simulink model "P8_Signal_Conditioning_Circuit"  (R2023b)
settings: Solver=FixedStepAuto  StartTime=0.0  StopTime=1  FixedStep=1e-6  RelTol=1e-9
libraries: spsSeriesRLCBranchLib x23, spsVoltageMeasurementLib x15, spsGroundLib x14, spsDiodeLib x9, spsControlledVoltageSourceLib x5, simulink x4, spsACVoltageSourceLib x2, spsIdealSwitchLib x1, eePwmGenerator x1, spsDCVoltageSourceLib x1, sps_lib x1
settings Model: Creator=Lucas  LastModifiedBy=Lucas

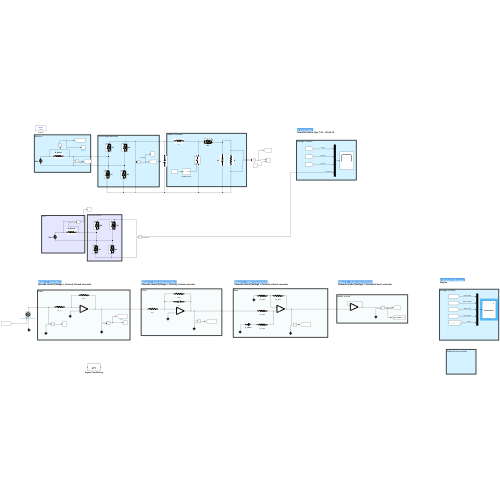
[thumbnail: Simulink's stored preview of the top-level diagram]
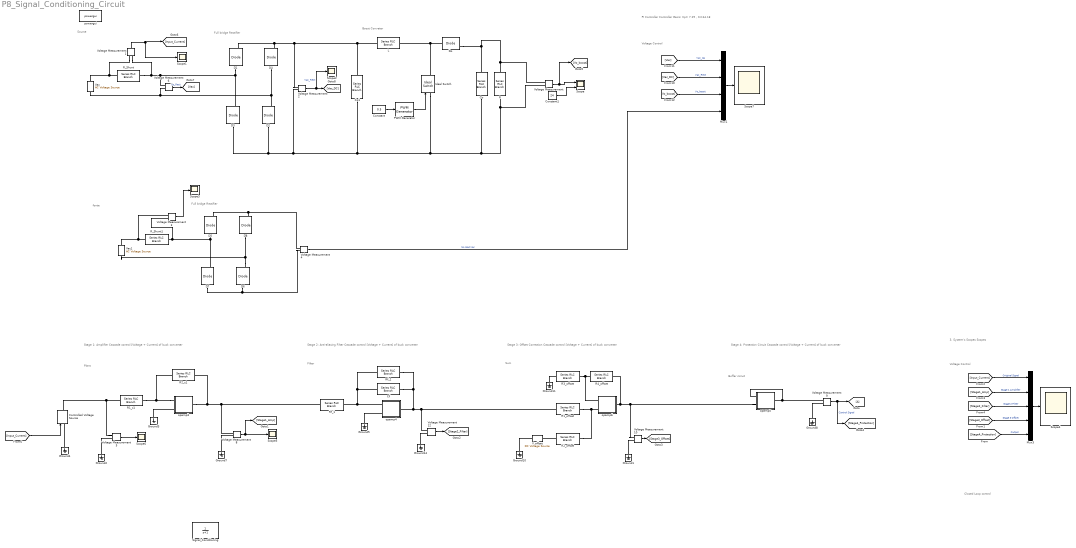
== system P8_Signal_Conditioning_Circuit ==
  note: Boost Conveter
  note: Full bridge Rectifier
  note: Source
  note: Full bridge Rectifier
  note: fonte
  note: PI Controller
      | Controller Gains: Kp= 7.29 , Ki=44.18
  note: Stage 1: Amplifier
      | Cascade control [Voltage + Current] of buck converter
  note: Stage 2: Anti-aliasing Filter
      | Cascade control [Voltage + Current] of buck converter
  note: Stage 3: Offset Correction
      | Cascade control [Voltage + Current] of buck converter
  note: Stage 4: Protection Circuit
      | Cascade control [Voltage + Current] of buck converter
  note: Closed Loop control
  note: Plant
  note: Voltage Control
  note: 3. System's Scopes
      | Scopes
  note: Filter
  note: Sum
  note: Buffer circuit
  note: Voltage Control
  Cf : spsSeriesRLCBranchLib/Series RLC Branch  LConnTagsString=__new0  RConnTagsString=__new0  BranchType=C  Resistance=1e3  Inductance=1e-3  SetiL0=off  InitialCurrent=0  Capacitance=4.9e-9  Setx0=off  InitialVoltage=0  Measurements=None
  Co : spsSeriesRLCBranchLib/Series RLC Branch  LConnTagsString=__new0  RConnTagsString=__new0  BranchType=C  Resistance=1  Inductance=1e-3  SetiL0=off  InitialCurrent=0  Capacitance=510e-6  Setx0=off  InitialVoltage=0  Measurements=None
  Co1 : spsSeriesRLCBranchLib/Series RLC Branch  LConnTagsString=__new0  RConnTagsString=__new0  BranchType=C  Resistance=1  Inductance=1e-3  SetiL0=off  InitialCurrent=0  Capacitance=1  Setx0=off  InitialVoltage=0  Measurements=None
  Constant : Constant  Value=0.5
  Constant1 : Constant  Value=24
  Controlled Voltage Source : spsControlledVoltageSourceLib/Controlled Voltage Source  Initialize=on  Source_Type=AC  Amplitude=0  Phase=0  Frequency=0  Measurements=None
  D{1..8} (8 alike) : spsDiodeLib/Diode  Ron=0.001  Lon=0  Vf=0  IC=0  UseSnubber=0  Rs=500  Cs=250e-9  Measurements=on
  Do : spsDiodeLib/Diode  Ron=0.001  Lon=0  Vf=0  IC=0  UseSnubber=0  Rs=500  Cs=250e-9  Measurements=on
  Goto : Goto
  Ground{1..5,7..8,10..11,14} (10 alike) : spsGroundLib/Ground  LConnTagsString=a
  Ideal Switch : spsIdealSwitchLib/Ideal Switch  Ron=0.001  Lon=0  IC=0  Rs=inf  Cs=inf  Measurements=on
  L : spsSeriesRLCBranchLib/Series RLC Branch  LConnTagsString=__new0  RConnTagsString=__new0  BranchType=L  Resistance=1  Inductance=100e-3  SetiL0=off  InitialCurrent=0  Capacitance=1e-6  Setx0=off  InitialVoltage=0  Measurements=None
  Mux1 : Mux
  Mux3 : Mux  Inputs=5
  PWM Generator : eePwmGenerator/PWM Generator  CarrCount=Up  Tper=1/(80e3)  Tdelay=0  Ts=1e-6
  R : spsSeriesRLCBranchLib/Series RLC Branch  LConnTagsString=__new0  RConnTagsString=__new0  BranchType=R  Resistance=10  Inductance=1e-3  SetiL0=off  InitialCurrent=0  Capacitance=1e-6  Setx0=off  InitialVoltage=0  Measurements=None
  R1_c1 : spsSeriesRLCBranchLib/Series RLC Branch  LConnTagsString=__new0  RConnTagsString=__new0  BranchType=R  Resistance=4e3  Inductance=1e-3  SetiL0=off  InitialCurrent=0  Capacitance=1e-6  Setx0=off  InitialVoltage=0  Measurements=None
  R1_offset : spsSeriesRLCBranchLib/Series RLC Branch  LConnTagsString=__new0  RConnTagsString=__new0  BranchType=R  Resistance=10e3  Inductance=1e-3  SetiL0=off  InitialCurrent=0  Capacitance=1e-6  Setx0=off  InitialVoltage=0  Measurements=None
  R2_c1 : spsSeriesRLCBranchLib/Series RLC Branch  LConnTagsString=__new0  RConnTagsString=__new0  BranchType=R  Resistance=1e3  Inductance=1e-3  SetiL0=off  InitialCurrent=0  Capacitance=1e-6  Setx0=off  InitialVoltage=0  Measurements=None
  R2_offset : spsSeriesRLCBranchLib/Series RLC Branch  LConnTagsString=__new0  RConnTagsString=__new0  BranchType=R  Resistance=10e3  Inductance=1e-3  SetiL0=off  InitialCurrent=0  Capacitance=1e-6  Setx0=off  InitialVoltage=0  Measurements=None
  R3_offset : spsSeriesRLCBranchLib/Series RLC Branch  LConnTagsString=__new0  RConnTagsString=__new0  BranchType=R  Resistance=10e3  Inductance=1e-3  SetiL0=off  InitialCurrent=0  Capacitance=1e-6  Setx0=off  InitialVoltage=0  Measurements=None
  R4_offset : spsSeriesRLCBranchLib/Series RLC Branch  LConnTagsString=__new0  RConnTagsString=__new0  BranchType=R  Resistance=10e3  Inductance=1e-3  SetiL0=off  InitialCurrent=0  Capacitance=1e-6  Setx0=off  InitialVoltage=0  Measurements=None
  R_Shunt : spsSeriesRLCBranchLib/Series RLC Branch  LConnTagsString=__new0  RConnTagsString=__new0  BranchType=R  Resistance=0.1  Inductance=1e-3  SetiL0=off  InitialCurrent=0  Capacitance=1e-6  Setx0=off  InitialVoltage=0  Measurements=None
  R_Shunt1 : spsSeriesRLCBranchLib/Series RLC Branch  LConnTagsString=__new0  RConnTagsString=__new0  BranchType=R  Resistance=0.1  Inductance=1e-3  SetiL0=off  InitialCurrent=0  Capacitance=1e-6  Setx0=off  InitialVoltage=0  Measurements=None
  Rf_1 : spsSeriesRLCBranchLib/Series RLC Branch  LConnTagsString=__new0  RConnTagsString=__new0  BranchType=R  Resistance=1e3  Inductance=1e-3  SetiL0=off  InitialCurrent=0  Capacitance=1e-6  Setx0=off  InitialVoltage=0  Measurements=None
  Rf_2 : spsSeriesRLCBranchLib/Series RLC Branch  LConnTagsString=__new0  RConnTagsString=__new0  BranchType=R  Resistance=1e3  Inductance=1e-3  SetiL0=off  InitialCurrent=0  Capacitance=1e-6  Setx0=off  InitialVoltage=0  Measurements=None
  Scope : Scope  NumInputPorts=2
  Scope{1..7} (7 alike) : Scope
  Signal_Conditioning : TransferFcn  Denominator=[1 1]
  V_offset : spsDCVoltageSourceLib/DC Voltage Source  Amplitude=2.5  Measurements=None
  Vac : spsACVoltageSourceLib/AC Voltage Source  Amplitude=12  Phase=0  Frequency=60  SampleTime=1e-6  Measurements=None  BusType=swing  Pref=10e3  Qref=0  Qmin=-inf  Qmax=+inf
  Vac1 : spsACVoltageSourceLib/AC Voltage Source  Amplitude=12  Phase=0  Frequency=60  SampleTime=0  Measurements=None  BusType=swing  Pref=10e3  Qref=0  Qmin=-inf  Qmax=+inf
  Voltage Measurement{,1..6,8..10,12} (11 alike) : spsVoltageMeasurementLib/Voltage Measurement  PhasorSimulation=off  OutputType=Complex  PSBequivalent=0
  opamp3 : Subsystem  mask(Opamp){Ri=1e7, Ro=100, A=200000, U1=15, U2=-15}
      mask prompts: Ri "Input Resistance"; Ro "Output Resistance"; A "Open loop amplification"; U1 "Upper limit supply voltage"; U2 "Lower limit supply voltage"
      mask Display:
      | plot([10 20 30 40], [10 12 14 16],[10 20 30 40], [22 20 18 16],[10 10],[10 22])
      | text(10,13.4,'+')
      | text(10,21,'_')
  opamp4 : Subsystem  mask(Opamp){Ri=1e7, Ro=100, A=200000, U1=15, U2=-15}
      mask prompts: Ri "Input Resistance"; Ro "Output Resistance"; A "Open loop amplification"; U1 "Upper limit supply voltage"; U2 "Lower limit supply voltage"
      mask Display:
      | plot([10 20 30 40], [10 12 14 16],[10 20 30 40], [22 20 18 16],[10 10],[10 22])
      | text(10,13.4,'+')
      | text(10,21,'_')
  opamp5 : Subsystem  mask(Opamp){Ri=1e7, Ro=100, A=200000, U1=5, U2=0}
      mask prompts: Ri "Input Resistance"; Ro "Output Resistance"; A "Open loop amplification"; U1 "Upper limit supply voltage"; U2 "Lower limit supply voltage"
      mask Display:
      | plot([10 20 30 40], [10 12 14 16],[10 20 30 40], [22 20 18 16],[10 10],[10 22])
      | text(10,13.4,'+')
      | text(10,21,'_')
  opamp6 : Subsystem  mask(Opamp){Ri=1e7, Ro=100, A=200000, U1=15, U2=-15}
      mask prompts: Ri "Input Resistance"; Ro "Output Resistance"; A "Open loop amplification"; U1 "Upper limit supply voltage"; U2 "Lower limit supply voltage"
      mask Display:
      | plot([10 20 30 40], [10 12 14 16],[10 20 30 40], [22 20 18 16],[10 10],[10 22])
      | text(10,13.4,'+')
      | text(10,21,'_')
  powergui : sps_lib/powergui  Priority=1  SimulationMode=Discrete  SampleTime=1e-6  frequency=60  Iterations=50  frequencyindice=0  Pbase=100e6  ErrMax=1e-4  UnitsV=kV  UnitsW=MW  buscounter=0  FunctionMessages=off  echomessages=off  EnableUseOfTLC=off  CurrentSourceSwitches=off  DisableSnubberDevices=off  DisableRonSwitches=off  DisableVfSwitches=off  DisplayEquations=off  AutomaticDiscreteSolvers=off  SolverType=Tustin/Backward Euler (TBE)  Interpol=off  ExternalGateDelay=off  methode=off  Ts=100  x0status=blocks  SPID=on  SwTol=0  HookPort=off  NonlinearTolerance=1e-4  nMaxIteration=100  ContinueOnMaxIteration=off  RestoreLinks=warning  ResistiveCurrentMeasurement=off  Frange=[0:2:500]  Ylog=off  Xlog=on  ShowGrid=off  save=off  variable=ZData  structure=0  ZoomFFT=off  StartTime=0.0  cycles=1  DisplayStyle=1  fundamental=60  FreqAxis=off  MaxFrequency=1000  frequencyindicesteady=1  RmsSteady=1  display=off
  wires:
  Constant/1 -> PWM Generator/1
  PWM Generator/1 -> Ideal Switch/1
  Voltage Measurement/1 -> [Vo_boost], Scope/1
  Voltage Measurement1/1 -> Scope1/1, [Input_Current]
  Voltage Measurement2/1 -> [Vac_DC], Scope2/1  "Vac_Rect"
  Voltage Measurement3/1 -> Scope3/1
  Constant1/1 -> Scope/2
  Voltage Measurement8/1 -> Scope5/1, [Stage1_Amp]
  Voltage Measurement9/1 -> [Stage4_Protection], Goto/1  "Control Signal"
  [Input_Current] -> Mux3/1  "Original Signal"
  [Stage4_Protection] -> Mux3/5  "Output"
  [Stage3_Offset] -> Mux3/4  "Stage 3 Offset"
  [Stage2_Filter] -> Mux3/3  "Stage 2 Filter"
  Mux3/1 -> Scope4/1
  Voltage Measurement5/1 -> Scope6/1
  Voltage Measurement12/1 -> [Stage2_Filter]
  Voltage Measurement10/1 -> [Stage3_Offset]
  [Stage1_Amp] -> Mux3/2  "Stage 1 Amplifier"
  Voltage Measurement6/1 -> [Vac]  "Vo_Rect"
  [Vo_boost] -> Mux1/3  "Vo_boost"
  Mux1/1 -> Scope7/1
  [Vac] -> Mux1/1  "Vac_og"
  [Vac_DC] -> Mux1/2  "Vac_Rect"
  [Input_Current] -> Controlled Voltage Source/1
  Voltage Measurement4/1 -> Mux1/4  "No load Vac"
  connections:
  D1/LConn1 -- Voltage Measurement6/LConn1 -- Voltage Measurement1/LConn2 -- R_Shunt/RConn1 -- D3/RConn1
  D4/LConn1 -- Voltage Measurement6/LConn2 -- Vac/LConn1 -- D2/RConn1
  D4/RConn1 -- L/LConn1 -- Co1/LConn1 -- Voltage Measurement2/LConn1 -- D1/RConn1
  Do/LConn1 -- L/RConn1 -- Ideal Switch/RConn1
  R/RConn1 -- Voltage Measurement/LConn1 -- Co/LConn1 -- Do/RConn1
  Co/RConn1 -- Ideal Switch/LConn1 -- Voltage Measurement2/LConn2 -- D2/LConn1 -- D3/LConn1 -- Co1/RConn1 -- R/LConn1 -- Voltage Measurement/LConn2
  R_Shunt/LConn1 -- Voltage Measurement1/LConn1 -- Vac/RConn1
  D6/RConn1 -- D8/LConn1 -- Vac1/LConn1
  Voltage Measurement3/LConn1 -- R_Shunt1/LConn1 -- Vac1/RConn1
  D8/RConn1 -- D5/RConn1 -- Voltage Measurement4/LConn1
  D7/LConn1 -- Voltage Measurement4/LConn2 -- D6/LConn1
  Voltage Measurement3/LConn2 -- D7/RConn1 -- D5/LConn1 -- R_Shunt1/RConn1
  R1_offset/LConn1 -- Voltage Measurement12/LConn1 -- Rf_2/RConn1 -- Cf/RConn1 -- opamp4/RConn1
  Rf_1/RConn1 -- Cf/LConn1 -- Rf_2/LConn1 -- opamp4/LConn1
  Voltage Measurement8/LConn1 -- Rf_1/LConn1 -- opamp3/RConn1 -- R2_c1/RConn1
  opamp3/LConn1 -- R1_c1/RConn1 -- R2_c1/LConn1
  opamp3/LConn2 -- Ground3/LConn1
  opamp4/LConn2 -- Ground5/LConn1
  Ground7/LConn1 -- Voltage Measurement8/LConn2
  opamp5/LConn1 -- opamp5/RConn1 -- Voltage Measurement9/LConn1
  Ground8/LConn1 -- Voltage Measurement9/LConn2
  R3_offset/RConn1 -- R4_offset/LConn1 -- opamp6/LConn1
  Voltage Measurement10/LConn1 -- opamp5/LConn2 -- opamp6/RConn1 -- R4_offset/RConn1
  Ground10/LConn1 -- V_offset/LConn1
  R3_offset/LConn1 -- Ground11/LConn1
  R1_offset/RConn1 -- R2_offset/RConn1 -- opamp6/LConn2
  R2_offset/LConn1 -- V_offset/RConn1
  Ground14/LConn1 -- Voltage Measurement12/LConn2
  Ground1/LConn1 -- Voltage Measurement10/LConn2
  Ground2/LConn1 -- Voltage Measurement5/LConn2
  Voltage Measurement5/LConn1 -- R1_c1/LConn1 -- Controlled Voltage Source/RConn1
  Ground4/LConn1 -- Controlled Voltage Source/LConn1

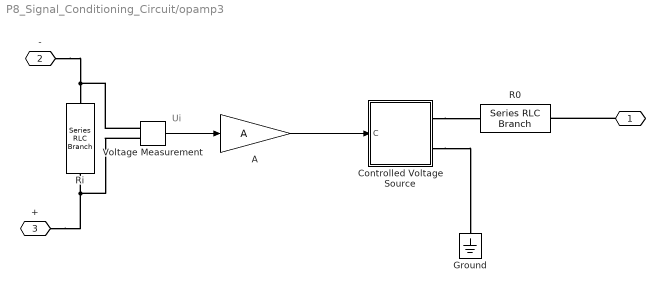
== system P8_Signal_Conditioning_Circuit/opamp3 ==
  note: Ui
  A : Gain  Gain=A
  Controlled Voltage Source : Subsystem
  Ground : spsGroundLib/Ground  LConnTagsString=a
  R0 : spsSeriesRLCBranchLib/Series RLC Branch  LConnTagsString=__new0  RConnTagsString=__new0  BranchType=R  Resistance=Ro  Inductance=1.0  SetiL0=off  InitialCurrent=0  Capacitance=1.0  Setx0=off  InitialVoltage=0  Measurements=None
  Ri : spsSeriesRLCBranchLib/Series RLC Branch  LConnTagsString=__new0  RConnTagsString=__new0  BranchType=R  Resistance=Ri  Inductance=1.0  SetiL0=off  InitialCurrent=0  Capacitance=1.0  Setx0=off  InitialVoltage=0  Measurements=None
  Voltage Measurement : spsVoltageMeasurementLib/Voltage Measurement  PhasorSimulation=off  OutputType=Complex  PSBequivalent=0
  " " : PMIOPort  Side=Right
  - : PMIOPort  Port=2  Side=Left
  + : PMIOPort  Port=3  Side=Left
  wires:
  Voltage Measurement/1 -> A/1
  A/1 -> Controlled Voltage Source/1(C)
  connections:
  " "/RConn1 -- R0/LConn1
  Controlled Voltage Source/RConn1 -- R0/RConn1
  -/RConn1 -- Voltage Measurement/LConn1 -- Ri/LConn1
  +/RConn1 -- Voltage Measurement/LConn2 -- Ri/RConn1
  Controlled Voltage Source/RConn2 -- Ground/LConn1

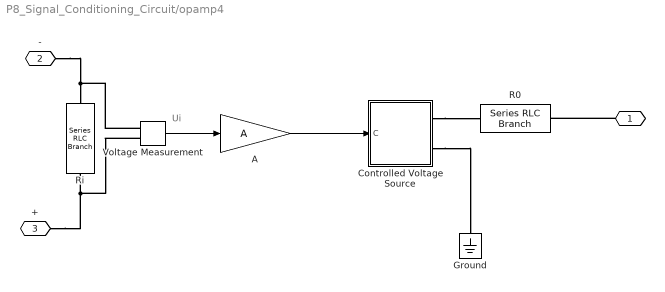
== system P8_Signal_Conditioning_Circuit/opamp4 ==
  note: Ui
  A : Gain  Gain=A
  Controlled Voltage Source : Subsystem
  Ground : spsGroundLib/Ground  LConnTagsString=a
  R0 : spsSeriesRLCBranchLib/Series RLC Branch  LConnTagsString=__new0  RConnTagsString=__new0  BranchType=R  Resistance=Ro  Inductance=1.0  SetiL0=off  InitialCurrent=0  Capacitance=1.0  Setx0=off  InitialVoltage=0  Measurements=None
  Ri : spsSeriesRLCBranchLib/Series RLC Branch  LConnTagsString=__new0  RConnTagsString=__new0  BranchType=R  Resistance=Ri  Inductance=1.0  SetiL0=off  InitialCurrent=0  Capacitance=1.0  Setx0=off  InitialVoltage=0  Measurements=None
  Voltage Measurement : spsVoltageMeasurementLib/Voltage Measurement  PhasorSimulation=off  OutputType=Complex  PSBequivalent=0
  " " : PMIOPort  Side=Right
  - : PMIOPort  Port=2  Side=Left
  + : PMIOPort  Port=3  Side=Left
  wires:
  Voltage Measurement/1 -> A/1
  A/1 -> Controlled Voltage Source/1(C)
  connections:
  " "/RConn1 -- R0/LConn1
  Controlled Voltage Source/RConn1 -- R0/RConn1
  -/RConn1 -- Voltage Measurement/LConn1 -- Ri/LConn1
  +/RConn1 -- Voltage Measurement/LConn2 -- Ri/RConn1
  Controlled Voltage Source/RConn2 -- Ground/LConn1

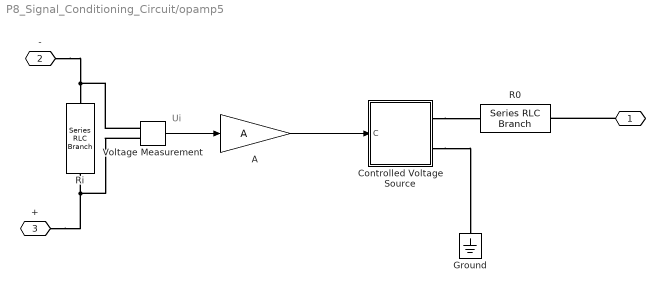
== system P8_Signal_Conditioning_Circuit/opamp5 ==
  note: Ui
  A : Gain  Gain=A
  Controlled Voltage Source : Subsystem
  Ground : spsGroundLib/Ground  LConnTagsString=a
  R0 : spsSeriesRLCBranchLib/Series RLC Branch  LConnTagsString=__new0  RConnTagsString=__new0  BranchType=R  Resistance=Ro  Inductance=1.0  SetiL0=off  InitialCurrent=0  Capacitance=1.0  Setx0=off  InitialVoltage=0  Measurements=None
  Ri : spsSeriesRLCBranchLib/Series RLC Branch  LConnTagsString=__new0  RConnTagsString=__new0  BranchType=R  Resistance=Ri  Inductance=1.0  SetiL0=off  InitialCurrent=0  Capacitance=1.0  Setx0=off  InitialVoltage=0  Measurements=None
  Voltage Measurement : spsVoltageMeasurementLib/Voltage Measurement  PhasorSimulation=off  OutputType=Complex  PSBequivalent=0
  " " : PMIOPort  Side=Right
  - : PMIOPort  Port=2  Side=Left
  + : PMIOPort  Port=3  Side=Left
  wires:
  Voltage Measurement/1 -> A/1
  A/1 -> Controlled Voltage Source/1(C)
  connections:
  " "/RConn1 -- R0/LConn1
  Controlled Voltage Source/RConn1 -- R0/RConn1
  -/RConn1 -- Voltage Measurement/LConn1 -- Ri/LConn1
  +/RConn1 -- Voltage Measurement/LConn2 -- Ri/RConn1
  Controlled Voltage Source/RConn2 -- Ground/LConn1

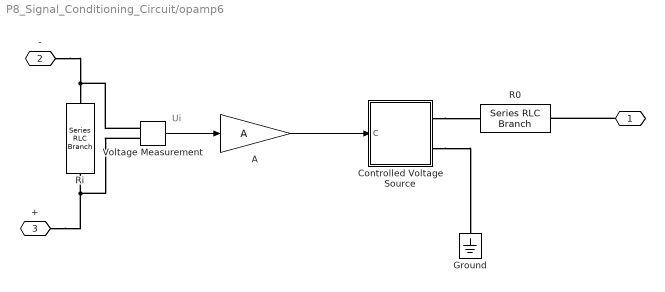
== system P8_Signal_Conditioning_Circuit/opamp6 ==
  note: Ui
  A : Gain  Gain=A
  Controlled Voltage Source : Subsystem
  Ground : spsGroundLib/Ground  LConnTagsString=a
  R0 : spsSeriesRLCBranchLib/Series RLC Branch  LConnTagsString=__new0  RConnTagsString=__new0  BranchType=R  Resistance=Ro  Inductance=1.0  SetiL0=off  InitialCurrent=0  Capacitance=1.0  Setx0=off  InitialVoltage=0  Measurements=None
  Ri : spsSeriesRLCBranchLib/Series RLC Branch  LConnTagsString=__new0  RConnTagsString=__new0  BranchType=R  Resistance=Ri  Inductance=1.0  SetiL0=off  InitialCurrent=0  Capacitance=1.0  Setx0=off  InitialVoltage=0  Measurements=None
  Voltage Measurement : spsVoltageMeasurementLib/Voltage Measurement  PhasorSimulation=off  OutputType=Complex  PSBequivalent=0
  " " : PMIOPort  Side=Right
  - : PMIOPort  Port=2  Side=Left
  + : PMIOPort  Port=3  Side=Left
  wires:
  Voltage Measurement/1 -> A/1
  A/1 -> Controlled Voltage Source/1(C)
  connections:
  " "/RConn1 -- R0/LConn1
  Controlled Voltage Source/RConn1 -- R0/RConn1
  -/RConn1 -- Voltage Measurement/LConn1 -- Ri/LConn1
  +/RConn1 -- Voltage Measurement/LConn2 -- Ri/RConn1
  Controlled Voltage Source/RConn2 -- Ground/LConn1

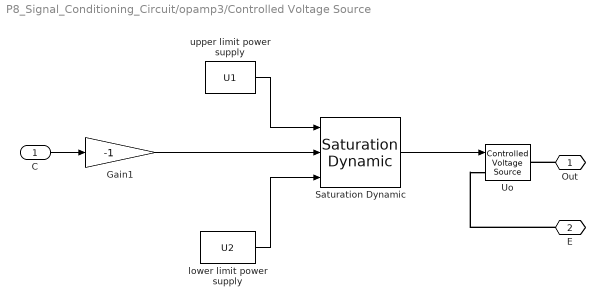
== system P8_Signal_Conditioning_Circuit/opamp3/Controlled Voltage Source ==
  C : Inport
  Gain1 : Gain  Gain=-1
  Saturation Dynamic : simulink/Discontinuities/Saturation Dynamic  OutMin=[]  OutMax=[]  OutDataTypeStr=Inherit: Same as second input  OutDataType=fixdt(1, 16)  OutScaling=2^-10  DoSatur=off
  Uo : spsControlledVoltageSourceLib/Controlled Voltage Source  Initialize=off  Source_Type=AC  Amplitude=0  Phase=0  Frequency=0  Measurements=None
  lower limit power supply : Constant  Value=U2
  upper limit power supply : Constant  Value=U1
  Out : PMIOPort  Side=Right
  E : PMIOPort  Port=2  Side=Right
  wires:
  Saturation Dynamic/1 -> Uo/1
  C/1 -> Gain1/1
  upper limit power supply/1 -> Saturation Dynamic/1
  lower limit power supply/1 -> Saturation Dynamic/3
  Gain1/1 -> Saturation Dynamic/2
  connections:
  E/RConn1 -- Uo/LConn1
  Out/RConn1 -- Uo/RConn1

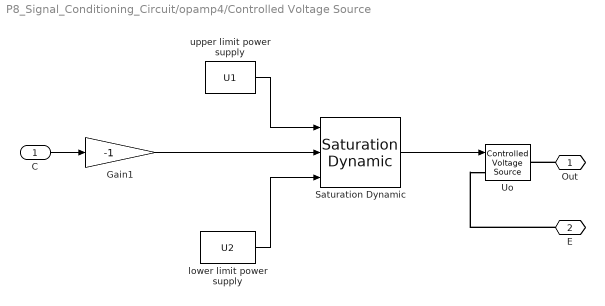
== system P8_Signal_Conditioning_Circuit/opamp4/Controlled Voltage Source ==
  C : Inport
  Gain1 : Gain  Gain=-1
  Saturation Dynamic : simulink/Discontinuities/Saturation Dynamic  OutMin=[]  OutMax=[]  OutDataTypeStr=Inherit: Same as second input  OutDataType=fixdt(1, 16)  OutScaling=2^-10  DoSatur=off
  Uo : spsControlledVoltageSourceLib/Controlled Voltage Source  Initialize=off  Source_Type=AC  Amplitude=0  Phase=0  Frequency=0  Measurements=None
  lower limit power supply : Constant  Value=U2
  upper limit power supply : Constant  Value=U1
  Out : PMIOPort  Side=Right
  E : PMIOPort  Port=2  Side=Right
  wires:
  Saturation Dynamic/1 -> Uo/1
  C/1 -> Gain1/1
  upper limit power supply/1 -> Saturation Dynamic/1
  lower limit power supply/1 -> Saturation Dynamic/3
  Gain1/1 -> Saturation Dynamic/2
  connections:
  E/RConn1 -- Uo/LConn1
  Out/RConn1 -- Uo/RConn1

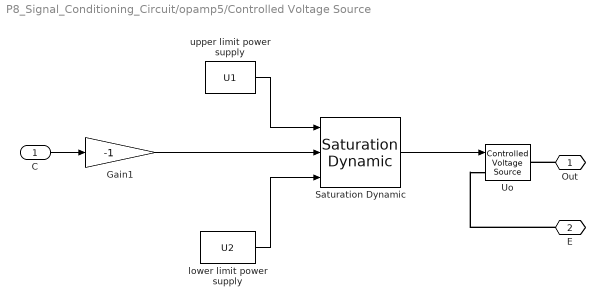
== system P8_Signal_Conditioning_Circuit/opamp5/Controlled Voltage Source ==
  C : Inport
  Gain1 : Gain  Gain=-1
  Saturation Dynamic : simulink/Discontinuities/Saturation Dynamic  OutMin=[]  OutMax=[]  OutDataTypeStr=Inherit: Same as second input  OutDataType=fixdt(1, 16)  OutScaling=2^-10  DoSatur=off
  Uo : spsControlledVoltageSourceLib/Controlled Voltage Source  Initialize=off  Source_Type=AC  Amplitude=0  Phase=0  Frequency=0  Measurements=None
  lower limit power supply : Constant  Value=U2
  upper limit power supply : Constant  Value=U1
  Out : PMIOPort  Side=Right
  E : PMIOPort  Port=2  Side=Right
  wires:
  Saturation Dynamic/1 -> Uo/1
  C/1 -> Gain1/1
  upper limit power supply/1 -> Saturation Dynamic/1
  lower limit power supply/1 -> Saturation Dynamic/3
  Gain1/1 -> Saturation Dynamic/2
  connections:
  E/RConn1 -- Uo/LConn1
  Out/RConn1 -- Uo/RConn1

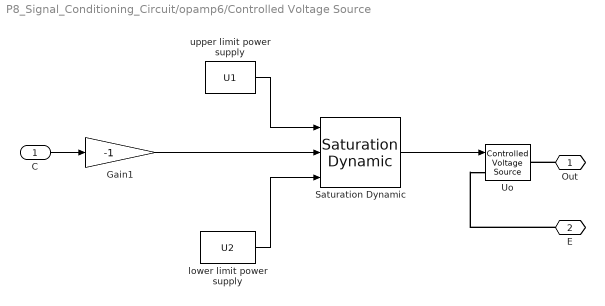
== system P8_Signal_Conditioning_Circuit/opamp6/Controlled Voltage Source ==
  C : Inport
  Gain1 : Gain  Gain=-1
  Saturation Dynamic : simulink/Discontinuities/Saturation Dynamic  OutMin=[]  OutMax=[]  OutDataTypeStr=Inherit: Same as second input  OutDataType=fixdt(1, 16)  OutScaling=2^-10  DoSatur=off
  Uo : spsControlledVoltageSourceLib/Controlled Voltage Source  Initialize=off  Source_Type=AC  Amplitude=0  Phase=0  Frequency=0  Measurements=None
  lower limit power supply : Constant  Value=U2
  upper limit power supply : Constant  Value=U1
  Out : PMIOPort  Side=Right
  E : PMIOPort  Port=2  Side=Right
  wires:
  Saturation Dynamic/1 -> Uo/1
  C/1 -> Gain1/1
  upper limit power supply/1 -> Saturation Dynamic/1
  lower limit power supply/1 -> Saturation Dynamic/3
  Gain1/1 -> Saturation Dynamic/2
  connections:
  E/RConn1 -- Uo/LConn1
  Out/RConn1 -- Uo/RConn1
